simulink model "stable2d"  (R2022a)
settings: Solver=FixedStepAuto  StartTime=0.0  StopTime=20  FixedStep=0.01  RelTol=1e-3
values from neighbouring files (symbols this model uses):
  x0 = 0.9 + X0(i,1)    [gen_data.m]
  y0 = -1.1 + X0(i,2)    [gen_data.m]
settings Model: Creator=diego  LastModifiedBy=diego

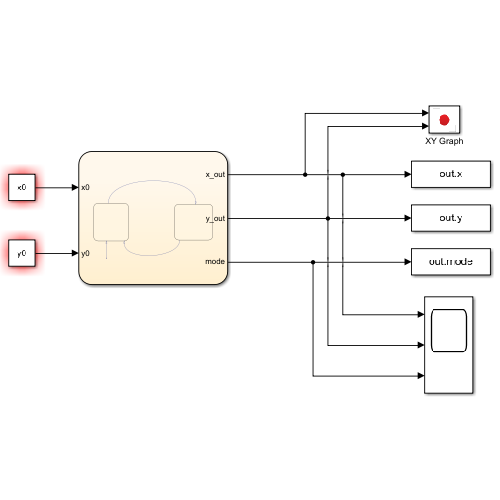
[thumbnail: Simulink's stored preview of the top-level diagram]
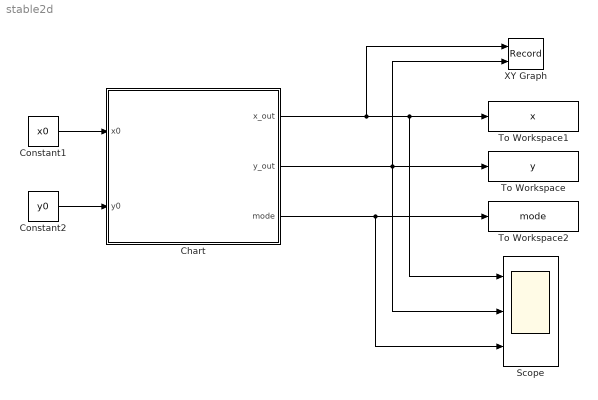
== system stable2d ==
  Chart : Stateflow chart  TreatAsAtomicUnit=on
  Constant1 : Constant  Value=x0
  Constant2 : Constant  Value=y0
  Scope : Scope  NumInputPorts=3
  To Workspace : ToWorkspace  VariableName=y  SampleTime=-1
  To Workspace1 : ToWorkspace  VariableName=x  SampleTime=-1
  To Workspace2 : ToWorkspace  VariableName=mode  SampleTime=-1
  XY Graph : Record  FileSettingsInternal="{\"entries\":[{\"content\":{\"excelSettings\":{\"content\":{},\"type\":\"Streamout.ExcelSettings\"}},\"type\":\"Streamout.FileSettingStorage\",\"uuid\":\"705d5765-8b1b-4c15-aebc-d8b422a4521f\"}],\"packageUris\":[\"http://schema.mathworks.com/mf0/streamout_blocks/R2020a\"],\"version\":\"1.0\"}"  Layout=[1 1]  SignalsInternal="{\"entries\":[{\"content\":{\"signals\":[{\"content\":{\"blockPath\":[\"stable2d/XY Graph\"],\"channel\":[],\"dimensions\":[1],\"domain\":\"stable2d/XY Graph\",\"lineColor\":\"#a2142f\",\"plots\":[1],\"port\":1,\"sid\":[\"\"],\"signalID\":869,\"signalName\":\"Chart:1\"},\"type\":\"RecordBlkView.Signal\",\"uuid\":\"0cb73176-13fe-4675-a623-b0837a9e0855\"},{\"content\":{\"blockPath\":[\"stable2d/XY Graph\"],\"channel\":[],\"dimensions\":[1],\"domain\":\"stable2d/XY Graph\",\"lineColor\":\"#139fff\",\"plots\":[1],\"port\":2,\"sid\":[\"\"],\"signalID\":873,\"signalName\":\"Chart:2\"},\"type\":\"RecordBlkView.Signal\",\"uuid\":\"5c124b1e-c8b9-4fee-b1ef-88f8e15f1d36\"}]},\"type\":\"RecordBlkView.InputSignals\",\"uuid\":\"a31ddcb3-ed69-4820-9913-7f8a0ad378e2\"}],\"packageUris\":[\"http://schema.mathworks.com/mf0/streamout_blocks/R2020a\"],\"version\":\"1.0\"}"  VisualizationBindings="{\"xyplotplugin\":{\"info\":[{\"series\":[{\"bindingParametersList\":[{\"parameter\":\"X-Axis\",\"signalID\":869,\"signalName\":\"Chart:1\"},{\"parameter\":\"Y-Axis\",\"signalID\":873,\"signalName\":\"Chart:2\"}],\"seriesID\":35679}],\"subplotID\":1}]}}"  CompatibilityTag=XY
  wires:
  Chart/1(x_out) -> XY Graph/1, Scope/1, To Workspace1/1
  Chart/2(y_out) -> Scope/2, To Workspace/1, XY Graph/2
  Constant1/1 -> Chart/1(x0)
  Constant2/1 -> Chart/2(y0)
  Chart/3(mode) -> Scope/3, To Workspace2/1

== stateflow chart stable2d/Chart ==
  settings: updateMethod=CONTINUOUS
  state Mode1
    du:
    x_dot = -y;
    y_dot = x^2;
    x_out = x;
    y_out = y;
    mode = 1;
  state Mode2
    du:
    x_dot = -y;
    y_dot = x^3;
    x_out = x;
    y_out = y;
    mode = 2;
  Mode1 -> Mode2 : [x-y < -3]
  Mode2 -> Mode1 : [y < -2]
  (default) -> Mode1 : {x = x0;
      | y = y0;}
  data: x_out output; y_out output; x local; y local; x0 input; y0 input; mode output
  data x settings: updateMethod=SF_CONTINUOUS_TIME_DATA
  data y settings: updateMethod=SF_CONTINUOUS_TIME_DATA
